simulink model "lab1_6"  (R2020a)
settings: Solver=VariableStepAuto  StartTime=0.0  StopTime=10.0  RelTol=1e-3
settings Model: Creator=huang  LastModifiedBy=huang

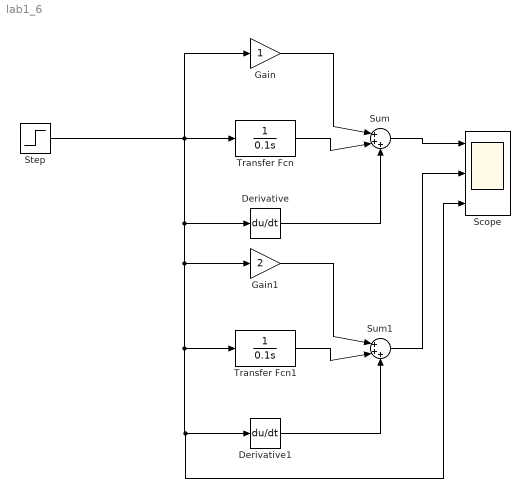
== system lab1_6 ==
  Derivative : Derivative  CoefficientInTFapproximation=0.1
  Derivative1 : Derivative  CoefficientInTFapproximation=0.02
  Gain : Gain
  Gain1 : Gain  Gain=2
  Scope : Scope  NumInputPorts=3
  Step : Step  Time=0  SampleTime=0
  Sum : Sum  Inputs=|+++
  Sum1 : Sum  Inputs=|+++
  Transfer Fcn : TransferFcn  Denominator=[0.1 0]
  Transfer Fcn1 : TransferFcn  Denominator=[0.1 0]
  wires:
  Gain/1 -> Sum/1
  Transfer Fcn/1 -> Sum/2
  Derivative/1 -> Sum/3
  Sum/1 -> Scope/1
  Sum1/1 -> Scope/2
  Derivative1/1 -> Sum1/3
  Transfer Fcn1/1 -> Sum1/2
  Gain1/1 -> Sum1/1
  Step/1 -> Transfer Fcn1/1, Scope/3, Derivative1/1, Gain1/1, Derivative/1, Gain/1, Transfer Fcn/1
